simulink model "PassengerVehicle"  (R2018b)
settings: configuration reference "Physics" (kept outside this file)
model workspace (MAT data in the model file):
  m = 1000
undefined symbols (not defined in the file): activate_Banking, activate_TrackProfile, P_BrakeGain, P_PassengerVehicleSimModel, P_SimFailureRearAxleGripStepEndTime_s, P_SimFailureRearAxleGripStepTime_s, POWTR__MODE__activate_ThrottleInterface, psi_rad, tireFR__MFSIMPLE__r_tire_m, tireRL__MFSIMPLE__r_tire_m, tSPhysics, VEH__ActuatorLimitation__deltaSteering_max_rad, VEH__ActuatorLimitation__deltaSteering_min_rad, VEH__ActuatorLimitation__Fx_Brake_max_N, VEH__ActuatorLimitation__Fx_Throttle_max_N, VEH__Brakes__BrakeBias_Front, VEH__Brakes__d_BrakeActuatorBoreFrRe_m__1, VEH__Brakes__d_BrakeActuatorBoreFrRe_m__2, VEH__Brakes__mue_BrakePadsFrRe_kinetic__1, VEH__Brakes__mue_BrakePadsFrRe_kinetic__2, VEH__Brakes__n_BrakePadsNumberFrRe__1, VEH__Brakes__n_BrakePadsNumberFrRe__2, VEH__Brakes__r_BrakePadsMeanLeverFrRe_m__1, VEH__Brakes__r_BrakePadsMeanLeverFrRe_m__2, VEH__Steering__T_Steering_s, VEH__VehicleData__l_WheelbaseF_m, VEH__VehicleData__l_WheelbaseTotal_m, VEH__VehicleData__w_TrackF_m, VEH__VehicleData__w_TrackR_m, x_m, y_m
libraries: general_sensor_lib x27, simulink x12
settings Model: DataDictionary=PassengerVehicle.sldd  PauseTimes=9.280  Creator=wischnewski  LastModifiedBy=ga25xiw

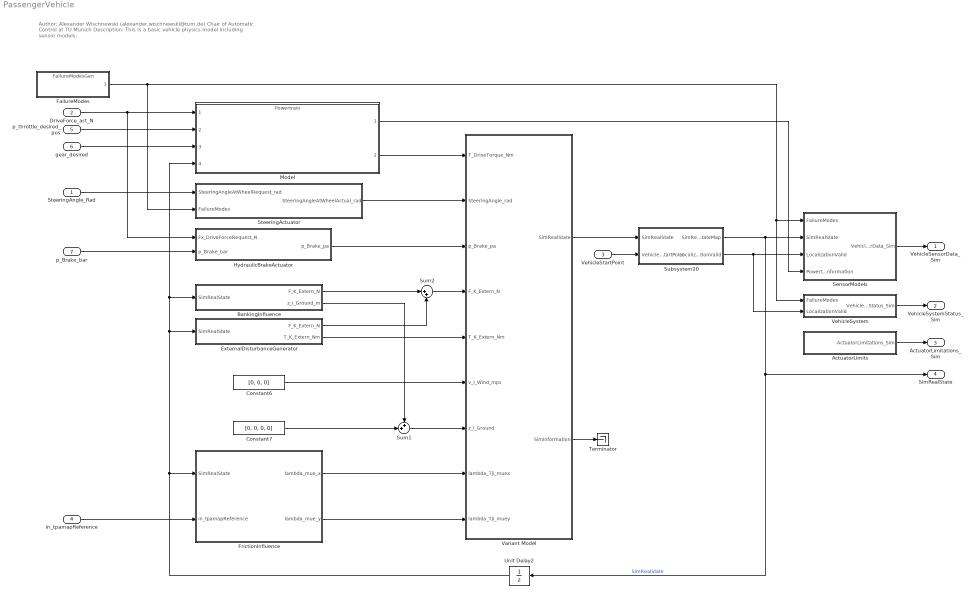
== system PassengerVehicle ==
  note: Author: Alexander Wischnewski (alexander.wischnewski@tum.de)
      | Chair of Automatic Control at TU Munich
      |
      | Description: This is a basic vehicle physics model including sensor models.
  SteeringAngle_Rad : Inport
  DriveForce_act_N : Inport  Port=2
  VehicleStartPoint : Inport  Port=3
  in_tpamapReference : Inport  Port=4  OutDataTypeStr=Bus: tpamapReference
  p_throttle_desired_pos : Inport  Port=5
  gear_desired : Inport  Port=6
  p_Brake_bar : Inport  Port=7
  ActuatorLimits : Subsystem
  BankingInfluence : Subsystem
  Constant6 : Constant  Value=[0, 0, 0]
  Constant7 : Constant  Value=[0, 0, 0, 0]
  ExternalDisturbanceGenerator : Subsystem
  FailureModes : ModelReference  ModelNameDialog=FailureModesGen  SimulationMode=Normal  ModelReferenceVersion=1.712
  FrictionInfluence : Subsystem
  HydraulicBrakeActuator : Subsystem
  Model : ModelReference  ModelNameDialog=Powertrain.slx  SimulationMode=Normal  ModelReferenceVersion=1.922
  SensorModels : Subsystem
  SteeringActuator : Subsystem
  Subsystem20 : Subsystem
  Sum1 : Sum  Inputs=++|
  Sum2 : Sum  Inputs=|++
  Terminator : Terminator
  Unit Delay2 : UnitDelay  SampleTime=-1
  Variant Model : Subsystem  Variant=on
  VehicleSystem : Subsystem
  VehicleSensorData_Sim : Outport  OutDataTypeStr=Bus: VehicleSensorData_Sim
  VehicleSystemStatus_Sim : Outport  Port=2  OutDataTypeStr=Bus: VehicleSystemStatus_Sim
  ActuatorLimitations_Sim : Outport  Port=3  OutDataTypeStr=Bus: ActuatorLimitations_Sim
  SimRealState : Outport  Port=4  OutDataTypeStr=Bus: SimRealState
  wires:
  FailureModes/1 -> SteeringActuator/2(FailureModes), VehicleSystem/1(FailureModes), SensorModels/1(FailureModes)
  SteeringActuator/1(SteeringAngleAtWheelActual_rad) -> Variant Model/2(SteeringAngle_rad)
  SensorModels/1(VehicleSensorData_Sim) -> VehicleSensorData_Sim/1
  Constant6/1 -> Variant Model/6(v_I_Wind_mps)
  VehicleSystem/1(VehicleSystemStatus_Sim) -> VehicleSystemStatus_Sim/1
  ActuatorLimits/1(ActuatorLimitations_Sim) -> ActuatorLimitations_Sim/1
  SteeringAngle_Rad/1 -> SteeringActuator/1(SteeringAngleAtWheelRequest_rad)
  HydraulicBrakeActuator/1(p_Brake_pa) -> Variant Model/3(p_Brake_pa)
  DriveForce_act_N/1 -> HydraulicBrakeActuator/1(Fx_DriveForceRequest_N), Model/1
  Model/2 -> Variant Model/1(T_DriveTorque_Nm)
  Subsystem20/1(SimRealStateMap) -> SensorModels/2(SimRealState), SimRealState/1, Unit Delay2/1  "SimRealState"
  VehicleStartPoint/1 -> Subsystem20/2(VehicleStartPoint)
  Subsystem20/2(LocalizationValid) -> VehicleSystem/2(LocalizationValid), SensorModels/3(LocalizationValid)
  Variant Model/1(SimRealState) -> Subsystem20/1(SimRealState)
  Variant Model/2(SimInformation) -> Terminator/1
  ExternalDisturbanceGenerator/2(T_K_Extern_Nm) -> Variant Model/5(T_K_Extern_Nm)
  ExternalDisturbanceGenerator/1(F_K_Extern_N) -> Sum2/2
  BankingInfluence/1(F_K_Extern_N) -> Sum2/1
  Sum2/1 -> Variant Model/4(F_K_Extern_N)
  Sum1/1 -> Variant Model/7(z_I_Ground)
  BankingInfluence/2(z_I_Ground_m) -> Sum1/1
  Constant7/1 -> Sum1/2
  FrictionInfluence/2(lambda_mue_y) -> Variant Model/9(lambda_Tji_muey)
  FrictionInfluence/1(lambda_mue_x) -> Variant Model/8(lambda_Tji_muex)
  in_tpamapReference/1 -> FrictionInfluence/2(in_tpamapReference)
  p_throttle_desired_pos/1 -> Model/2
  gear_desired/1 -> Model/3
  Model/1 -> SensorModels/4(PowertrainInformation)
  Unit Delay2/1 -> ExternalDisturbanceGenerator/1(SimRealState), Model/4, BankingInfluence/1(SimRealState), FrictionInfluence/1(SimRealState)
  p_Brake_bar/1 -> HydraulicBrakeActuator/2(p_Brake_bar)

== system PassengerVehicle/ActuatorLimits ==
  Bus Creator : BusCreator  Inputs=4  OutDataTypeStr=Bus: ActuatorLimitations_Sim
  Constant : Constant  Value=VEH__ActuatorLimitation__deltaSteering_max_rad
  Constant1 : Constant  Value=VEH__ActuatorLimitation__deltaSteering_min_rad
  Constant2 : Constant  Value=VEH__ActuatorLimitation__Fx_Throttle_max_N
  Constant3 : Constant  Value=VEH__ActuatorLimitation__Fx_Brake_max_N
  ActuatorLimitations_Sim : Outport
  wires:
  Bus Creator/1 -> ActuatorLimitations_Sim/1
  Constant/1 -> Bus Creator/1  "SteeringAngleMax_rad"
  Constant1/1 -> Bus Creator/2  "SteeringAngleMin_rad"
  Constant2/1 -> Bus Creator/3  "DriveForceMax_N"
  Constant3/1 -> Bus Creator/4  "DriveForceMin_N"

== system PassengerVehicle/BankingInfluence ==
  SimRealState : Inport  OutDataTypeStr=Bus: SimRealState
  Banking disabled : Subsystem  TreatAsAtomicUnit=on
  Banking enabled : Subsystem  TreatAsAtomicUnit=on
  Compare To Zero : simulink/Logic and Bit Operations/Compare To Zero  relop===  OutDataTypeStr=boolean
  Constant : Constant  Value=activate_Banking
  Merge : Subsystem
  F_K_Extern_N : Outport
  z_I_Ground_m : Outport  Port=2
  wires:
  SimRealState/1 -> Banking enabled/1(SimRealState), Banking disabled/1(SimRealState)
  Constant/1 -> Merge/3(In3), Compare To Zero/1, Banking enabled/Enable
  Compare To Zero/1 -> Banking disabled/Enable
  Banking enabled/1(F_K_Extern_N) -> Merge/1(In1)
  Banking enabled/2(z_I_Ground_m) -> Merge/2(In2)
  Banking disabled/1(F_K_Extern_N) -> Merge/4(In4)
  Banking disabled/2(z_I_Ground_m) -> Merge/5(In5)
  Merge/1(Out1) -> F_K_Extern_N/1
  Merge/2(Out2) -> z_I_Ground_m/1

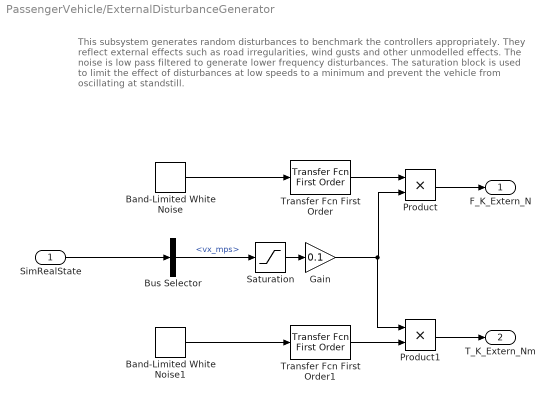
== system PassengerVehicle/ExternalDisturbanceGenerator ==
  note: This subsystem generates random disturbances to
      | benchmark the controllers appropriately. They reflect external effects
      | such as road irregularities, wind gusts and other unmodelled effects.
      |
      | The noise is low pass filtered to generate lower frequency disturbances.
      |
      | The saturation block is used to limit the effect of disturbances at low speeds to a minimum
      | and prevent the vehicle from oscillating at standstill.
  SimRealState : Inport
  Band-Limited White Noise : simulink/Sources/Band-Limited White Noise  Cov=[100^2 100^2 100^2]  Ts=tSPhysics  seed=[23341 325 10250]
  Band-Limited White Noise1 : simulink/Sources/Band-Limited White Noise  Cov=[25^2 25^2 25^2]  Ts=tSPhysics  seed=[456 7599 12475]
  Bus Selector : BusSelector  OutputSignals=vx_mps
  Gain : Gain  Gain=0.1
  Product : Product
  Product1 : Product
  Saturation : Saturate  UpperLimit=10  LowerLimit=0
  Transfer Fcn First Order : simulink/Discrete/Transfer Fcn First Order  PoleZ=0.99  ICPrevOutput=0.0  DoSatur=off
      settings: SourceProductName=Simulink
  Transfer Fcn First Order1 : simulink/Discrete/Transfer Fcn First Order  PoleZ=0.99  ICPrevOutput=0.0  DoSatur=off
      settings: SourceProductName=Simulink
  F_K_Extern_N : Outport
  T_K_Extern_Nm : Outport  Port=2
  wires:
  Band-Limited White Noise/1 -> Transfer Fcn First Order/1
  Band-Limited White Noise1/1 -> Transfer Fcn First Order1/1
  Transfer Fcn First Order/1 -> Product/1
  Product/1 -> F_K_Extern_N/1
  Transfer Fcn First Order1/1 -> Product1/2
  Product1/1 -> T_K_Extern_Nm/1
  Bus Selector/1 -> Saturation/1  "<vx_mps>"
  Saturation/1 -> Gain/1
  Gain/1 -> Product1/1, Product/2
  SimRealState/1 -> Bus Selector/1

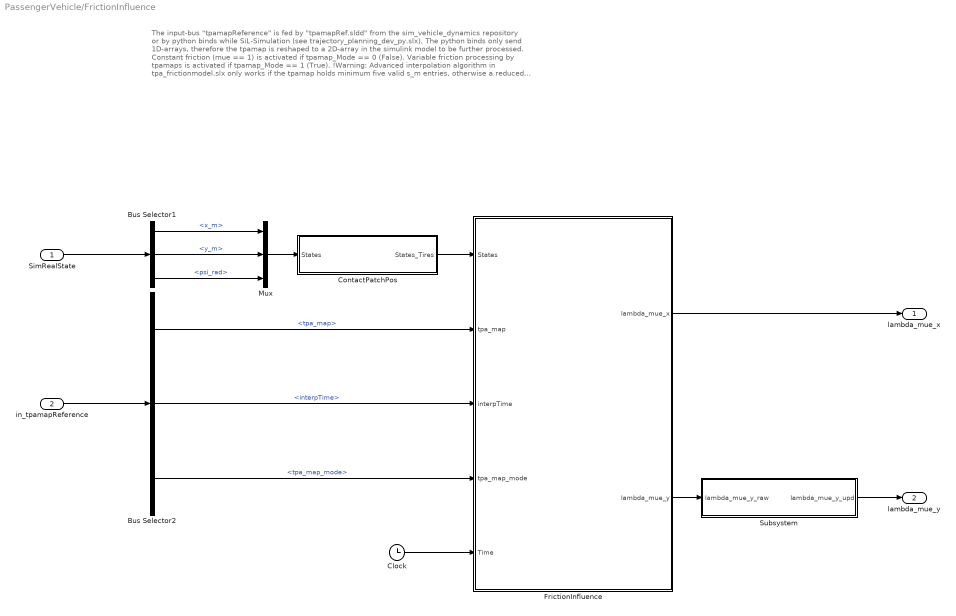
== system PassengerVehicle/FrictionInfluence ==
  note: The input-bus "tpamapReference" is fed by "tpamapRef.sldd" from the sim_vehicle_dynamics repository
      | or by python binds while SiL-Simulation (see trajectory_planning_dev_py.slx). The python binds only send
      | 1D-arrays, therefore the tpamap is reshaped to a 2D-array in the simulink model to be further processed.
      |
      | Constant friction (mue == 1) is activated if tpamap_Mode == 0 (False).
      | Variable friction processing by tpamaps is activated if tpamap_Mode == 1 (True).
      |
      | !Warning: Advanced interpolation algorithm in tpa_frictionmodel.slx only works if the tpamap holds minimum five valid s_m entries,
      |                 otherwise a reduced algorithm takes over, which assigns the local scaling factor of the nearest s_m entry to the lambda_mues
      |
      | Author: Dominik Stärk (dominik.staerk@tum.de)
  SimRealState : Inport
  in_tpamapReference : Inport  Port=2
  Bus Selector1 : BusSelector  OutputSignals=x_m,y_m,psi_rad
  Bus Selector2 : BusSelector  OutputSignals=tpa_map,interpTime,tpa_map_mode
  Clock : Clock
  ContactPatchPos : MATLAB Function  TreatAsAtomicUnit=on
  FrictionInfluence : MATLAB Function  TreatAsAtomicUnit=on
  Mux : Mux  Inputs=3
  Subsystem : Subsystem
  lambda_mue_x : Outport
  lambda_mue_y : Outport  Port=2
  wires:
  Bus Selector1/1 -> Mux/1  "<x_m>"
  Bus Selector1/2 -> Mux/2  "<y_m>"
  in_tpamapReference/1 -> Bus Selector2/1
  SimRealState/1 -> Bus Selector1/1
  Clock/1 -> FrictionInfluence/5(Time)
  Mux/1 -> ContactPatchPos/1(States)
  Bus Selector2/1 -> FrictionInfluence/2(tpa_map)  "<tpa_map>"
  Bus Selector2/2 -> FrictionInfluence/3(interpTime)  "<interpTime>"
  Bus Selector2/3 -> FrictionInfluence/4(tpa_map_mode)  "<tpa_map_mode>"
  FrictionInfluence/1(lambda_mue_x) -> lambda_mue_x/1
  Bus Selector1/3 -> Mux/3  "<psi_rad>"
  ContactPatchPos/1(States_Tires) -> FrictionInfluence/1(States)
  FrictionInfluence/2(lambda_mue_y) -> Subsystem/1(lambda_mue_y_raw)
  Subsystem/1(lambda_mue_y_upd) -> lambda_mue_y/1

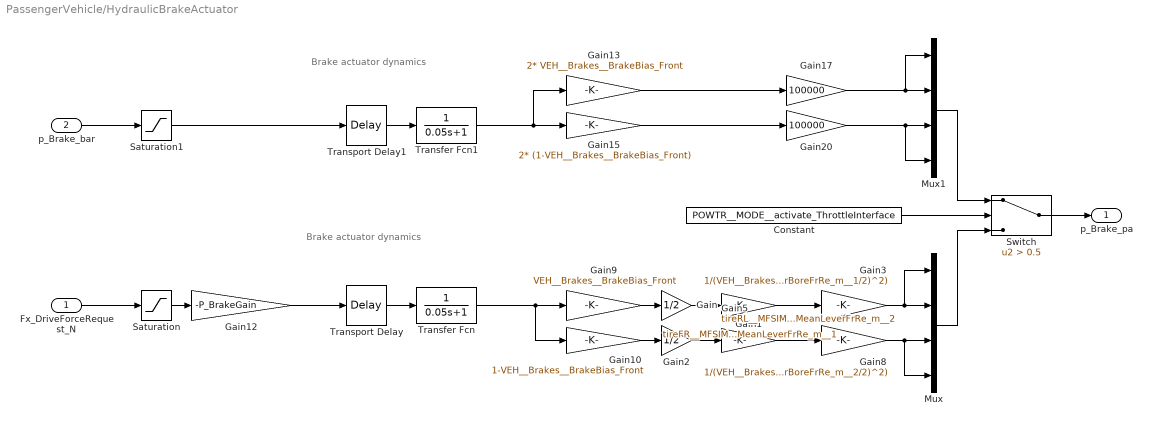
== system PassengerVehicle/HydraulicBrakeActuator ==
  note: Brake actuator dynamics
  note: Brake actuator dynamics
  Fx_DriveForceRequest_N : Inport
  p_Brake_bar : Inport  Port=2
  Constant : Constant  Value=POWTR__MODE__activate_ThrottleInterface
  Gain : Gain  Gain=1/2
  Gain1 : Gain  Gain=tireFR__MFSIMPLE__r_tire_m / VEH__Brakes__r_BrakePadsMeanLeverFrRe_m__1
  Gain10 : Gain  Gain=1-VEH__Brakes__BrakeBias_Front
  Gain12 : Gain  Gain=-P_BrakeGain
  Gain13 : Gain  Gain=2* VEH__Brakes__BrakeBias_Front
  Gain15 : Gain  Gain=2* (1-VEH__Brakes__BrakeBias_Front)
  Gain17 : Gain  Gain=100000
  Gain2 : Gain  Gain=1/2
  Gain20 : Gain  Gain=100000
  Gain3 : Gain  Gain=1/(VEH__Brakes__n_BrakePadsNumberFrRe__1*VEH__Brakes__mue_BrakePadsFrRe_kinetic__1*pi*(VEH__Brakes__d_BrakeActuatorBoreFrRe_m__1/2)^2)
  Gain5 : Gain  Gain=tireRL__MFSIMPLE__r_tire_m / VEH__Brakes__r_BrakePadsMeanLeverFrRe_m__2
  Gain8 : Gain  Gain=1/(VEH__Brakes__n_BrakePadsNumberFrRe__2*VEH__Brakes__mue_BrakePadsFrRe_kinetic__2*pi*(VEH__Brakes__d_BrakeActuatorBoreFrRe_m__2/2)^2)
  Gain9 : Gain  Gain=VEH__Brakes__BrakeBias_Front
  Mux : Mux
  Mux1 : Mux
  Saturation : Saturate  UpperLimit=0  LowerLimit=-inf
  Saturation1 : Saturate  UpperLimit=inf  LowerLimit=0
  Switch : Switch  Criteria=u2 > Threshold  Threshold=0.5
  Transfer Fcn : TransferFcn  Denominator=[0.05 1]
  Transfer Fcn1 : TransferFcn  Denominator=[0.05 1]
  Transport Delay : TransportDelay  DelayTime=0.02
  Transport Delay1 : TransportDelay  DelayTime=0.02
  p_Brake_pa : Outport
  wires:
  Gain8/1 -> Mux/3, Mux/4
  Gain3/1 -> Mux/1, Mux/2
  Fx_DriveForceRequest_N/1 -> Saturation/1
  Transfer Fcn/1 -> Gain10/1, Gain9/1
  Gain5/1 -> Gain8/1
  Gain1/1 -> Gain3/1
  Saturation/1 -> Gain12/1
  Transport Delay/1 -> Transfer Fcn/1
  Gain12/1 -> Transport Delay/1
  Constant/1 -> Switch/2
  p_Brake_bar/1 -> Saturation1/1
  Transport Delay1/1 -> Transfer Fcn1/1
  Saturation1/1 -> Transport Delay1/1
  Transfer Fcn1/1 -> Gain13/1, Gain15/1
  Gain13/1 -> Gain17/1
  Gain15/1 -> Gain20/1
  Mux1/1 -> Switch/1
  Mux/1 -> Switch/3
  Switch/1 -> p_Brake_pa/1
  Gain17/1 -> Mux1/1, Mux1/2
  Gain20/1 -> Mux1/4, Mux1/3
  Gain9/1 -> Gain/1
  Gain/1 -> Gain1/1
  Gain10/1 -> Gain2/1
  Gain2/1 -> Gain5/1

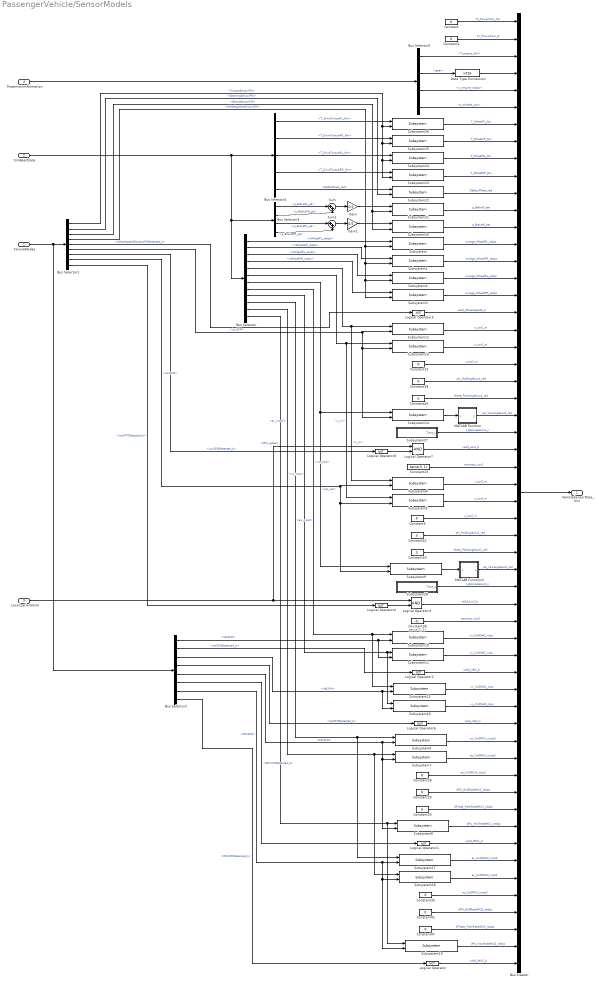
== system PassengerVehicle/SensorModels ==
  FailureModes : Inport
  SimRealState : Inport  Port=2
  LocalizationValid : Inport  Port=3
  PowertrainInformation : Inport  Port=4
  Bus Creator : BusCreator  Inputs=56  OutDataTypeStr=Bus: VehicleSensorData_Sim
  Bus Selector : BusSelector  OutputSignals=nWheelFL_radps,nWheelFR_radps,nWheelRL_radps,nWheelRR_radps,x_m,y_m,psi_rad,vx_mps,vy_mps,ax_mps2,ay_mps2,dPsi_radps
  Bus Selector1 : BusSelector  OutputSignals=TorqueSensorFM,SteeringSensorFM,BrakeSensorFM,WheelspeedSensorsFM,WheelspeedSensorsFMDetected_b,Loc1FM,Loc1FMDetected_b,Loc2FM,Loc2FMDetected_b
  Bus Selector2 : BusSelector  OutputSignals=Vel1FM,Vel1FMDetected_b,Vel2FM,Vel2FMDetected_b,IMU1FM,IMU1FMDetected_b,IMU2FM,IMU2FMDetected_b
  Bus Selector3 : BusSelector  OutputSignals=p_BrakeFL_pa,p_BrakeFR_pa,p_BrakeRL_pa,p_BrakeRR_pa
  Bus Selector4 : BusSelector  OutputSignals=T_DriveTorqueFL_Nm,T_DriveTorqueFR_Nm,T_DriveTorqueRL_Nm,T_DriveTorqueRR_Nm,DeltaWheel_rad
  Bus Selector5 : BusSelector  OutputSignals=T_engine_Nm,gear,w_engine_radps,p_throttle_pos
  Constant{,1,6,15,28..30,35,39..43,47} (14 alike) : Constant  Value=0
  Constant23 : Constant  Value=zeros(3, 1)
  Constant38 : Constant  Value=zeros(3, 1)
  Data Type Conversion : DataTypeConversion  OutDataTypeStr=int16
  Gain : Gain  Gain=0.5
  Gain1 : Gain  Gain=0.5
  Logical Operator{,1..2,4..6,8} (7 alike) : Logic  Operator=NOT  Inputs=1  AllPortsSameDT=off  OutDataTypeStr=boolean
  Logical Operator3 : Logic  AllPortsSameDT=off  OutDataTypeStr=boolean
  Logical Operator7 : Logic  AllPortsSameDT=off  OutDataTypeStr=boolean
  MATLAB Function : MATLAB Function  TreatAsAtomicUnit=on
  MATLAB Function2 : MATLAB Function  TreatAsAtomicUnit=on
  Subsystem : general_sensor_lib/Subsystem  Noise=0.1  Delay=0  SampleRate=tSPhysics  seed=436
  Subsystem1 : general_sensor_lib/Subsystem  Noise=0.1  Delay=0  SampleRate=tSPhysics  seed=438
  Subsystem10 : general_sensor_lib/Subsystem  Noise=0.01  Delay=0  SampleRate=tSPhysics  seed=4577
  Subsystem11 : general_sensor_lib/Subsystem  Noise=0.01  Delay=0  SampleRate=tSPhysics  seed=127
  Subsystem12 : general_sensor_lib/Subsystem  Noise=0.001  Delay=0  SampleRate=tSPhysics  seed=596
  Subsystem13 : general_sensor_lib/Subsystem  Noise=0.001  Delay=0  SampleRate=tSPhysics  seed=973
  Subsystem14 : general_sensor_lib/Subsystem  Noise=0.001  Delay=0  SampleRate=tSPhysics  seed=578
  Subsystem15 : general_sensor_lib/Subsystem  Noise=0.01  Delay=0  SampleRate=tSPhysics  seed=459
  Subsystem16 : general_sensor_lib/Subsystem  Noise=0.01  Delay=0  SampleRate=tSPhysics  seed=467
  Subsystem17 : general_sensor_lib/Subsystem  Noise=0.05  Delay=0  SampleRate=tSPhysics  seed=37
  Subsystem18 : general_sensor_lib/Subsystem  Noise=0.05  Delay=0  SampleRate=tSPhysics  seed=0
  Subsystem19 : general_sensor_lib/Subsystem  Noise=0.0002  Delay=0  SampleRate=tSPhysics  seed=0
  Subsystem2 : general_sensor_lib/Subsystem  Noise=0.1  Delay=0  SampleRate=tSPhysics  seed=137
  Subsystem20 : general_sensor_lib/Subsystem  Noise=1000000000  Delay=0  SampleRate=tSPhysics  seed=235
  Subsystem21 : general_sensor_lib/Subsystem  Noise=1000000000  Delay=0  SampleRate=tSPhysics  seed=798
  Subsystem22 : general_sensor_lib/Subsystem  Noise=1e-7  Delay=0  SampleRate=tSPhysics  seed=1234
  Subsystem23 : general_sensor_lib/Subsystem  Noise=100  Delay=0  SampleRate=tSPhysics  seed=438
  Subsystem24 : general_sensor_lib/Subsystem  Noise=100  Delay=0  SampleRate=tSPhysics  seed=368
  Subsystem25 : general_sensor_lib/Subsystem  Noise=100  Delay=0  SampleRate=tSPhysics  seed=978
  Subsystem26 : general_sensor_lib/Subsystem  Noise=100  Delay=0  SampleRate=tSPhysics  seed=138
  Subsystem27 : Subsystem
  Subsystem28 : Subsystem
  Subsystem3 : general_sensor_lib/Subsystem  Noise=0.1  Delay=0  SampleRate=tSPhysics  seed=345
  Subsystem4 : general_sensor_lib/Subsystem  Noise=0.001  Delay=0  SampleRate=tSPhysics  seed=596
  Subsystem5 : general_sensor_lib/Subsystem  Noise=0.001  Delay=0  SampleRate=tSPhysics  seed=973
  Subsystem6 : general_sensor_lib/Subsystem  Noise=0.05  Delay=0  SampleRate=tSPhysics  seed=456
  Subsystem7 : general_sensor_lib/Subsystem  Noise=0.05  Delay=0  SampleRate=tSPhysics  seed=78
  Subsystem8 : general_sensor_lib/Subsystem  Noise=0.0002  Delay=0  SampleRate=tSPhysics  seed=43
  Subsystem9 : general_sensor_lib/Subsystem  Noise=0.001  Delay=0  SampleRate=tSPhysics  seed=578
  Sum : Sum  Inputs=|++
  Sum1 : Sum  Inputs=|++
  VehicleSensorData_Sim : Outport
  wires:
  Bus Creator/1 -> VehicleSensorData_Sim/1
  Constant/1 -> Bus Creator/1  "Tz_Powertrain_Nm"
  Constant1/1 -> Bus Creator/2  "Fx_Powertrain_N"
  SimRealState/1 -> Bus Selector/1, Bus Selector3/1, Bus Selector4/1
  Bus Selector/1 -> Subsystem/1  "<nWheelFL_radps>"
  Bus Selector/2 -> Subsystem1/1  "<nWheelFR_radps>"
  Bus Selector/3 -> Subsystem2/1  "<nWheelRL_radps>"
  Bus Selector/4 -> Subsystem3/1  "<nWheelRR_radps>"
  Bus Selector/5 -> Subsystem4/1, Subsystem12/1  "<x_m>"
  Bus Selector/6 -> Subsystem5/1, Subsystem13/1  "<y_m>"
  Bus Selector/10 -> Subsystem17/1, Subsystem6/1  "<ax_mps2>"
  Bus Selector/11 -> Subsystem7/1, Subsystem18/1  "<ay_mps2>"
  Bus Selector/12 -> Subsystem19/1, Subsystem8/1  "<dPsi_radps>"
  Bus Selector/8 -> Subsystem15/1, Subsystem10/1  "<vx_mps>"
  Bus Selector/9 -> Subsystem16/1, Subsystem11/1  "<vy_mps>"
  Bus Selector/7 -> Subsystem9/1, Subsystem14/1  "<psi_rad>"
  FailureModes/1 -> Bus Selector1/1, Bus Selector2/1
  Bus Selector1/4 -> Subsystem/2, Subsystem1/2, Subsystem2/2, Subsystem3/2  "<WheelspeedSensorsFM>"
  Bus Selector1/5 -> Logical Operator5/1  "<WheelspeedSensorsFMDetected_b>"
  Bus Selector2/1 -> Subsystem11/2, Subsystem10/2  "<Vel1FM>"
  Bus Selector2/2 -> Logical Operator2/1  "<Vel1FMDetected_b>"
  Bus Selector2/5 -> Subsystem8/2, Subsystem7/2, Subsystem6/2  "<IMU1FM>"
  Bus Selector2/6 -> Logical Operator1/1  "<IMU1FMDetected_b>"
  Subsystem9/1 -> MATLAB Function2/1(u)
  Bus Selector2/3 -> Subsystem16/2, Subsystem15/2  "<Vel2FM>"
  Bus Selector2/4 -> Logical Operator6/1  "<Vel2FMDetected_b>"
  Bus Selector2/7 -> Subsystem19/2, Subsystem18/2, Subsystem17/2  "<IMU2FM>"
  Bus Selector2/8 -> Logical Operator/1  "<IMU2FMDetected_b>"
  Subsystem14/1 -> MATLAB Function/1(u)
  Logical Operator4/1 -> Logical Operator3/2
  Bus Selector1/9 -> Logical Operator4/1  "<Loc2FMDetected_b>"
  LocalizationValid/1 -> Logical Operator7/1, Logical Operator3/1
  Bus Selector1/8 -> Subsystem9/2, Subsystem5/2, Subsystem4/2  "<Loc2FM>"
  Bus Selector1/6 -> Subsystem14/2, Subsystem13/2, Subsystem12/2  "<Loc1FM>"
  Logical Operator8/1 -> Logical Operator7/2
  Bus Selector1/7 -> Logical Operator8/1  "<Loc1FMDetected_b>"
  Sum/1 -> Gain/1
  Sum1/1 -> Gain1/1
  Gain1/1 -> Subsystem20/1
  Gain/1 -> Subsystem21/1
  Bus Selector4/1 -> Subsystem26/1  "<T_DriveTorqueFL_Nm>"
  Bus Selector4/2 -> Subsystem25/1  "<T_DriveTorqueFR_Nm>"
  Bus Selector4/5 -> Subsystem22/1  "<DeltaWheel_rad>"
  Bus Selector3/1 -> Sum/1  "<p_BrakeFL_pa>"
  Bus Selector3/3 -> Sum1/1  "<p_BrakeRL_pa>"
  Bus Selector3/2 -> Sum/2  "<p_BrakeFR_pa>"
  Bus Selector3/4 -> Sum1/2  "<p_BrakeRR_pa>"
  Bus Selector4/4 -> Subsystem23/1  "<T_DriveTorqueRR_Nm>"
  Bus Selector4/3 -> Subsystem24/1  "<T_DriveTorqueRL_Nm>"
  Bus Selector1/3 -> Subsystem21/2, Subsystem20/2  "<BrakeSensorFM>"
  Bus Selector1/2 -> Subsystem22/2  "<SteeringSensorFM>"
  Bus Selector1/1 -> Subsystem23/2, Subsystem24/2, Subsystem25/2, Subsystem26/2  "<TorqueSensorFM>"
  PowertrainInformation/1 -> Bus Selector5/1
  Bus Selector5/1 -> Bus Creator/3  "<T_engine_Nm>"
  Bus Selector5/2 -> Data Type Conversion/1  "<gear>"
  Bus Selector5/3 -> Bus Creator/5  "<w_engine_radps>"
  Bus Selector5/4 -> Bus Creator/6  "<p_throttle_pos>"
  Subsystem26/1 -> Bus Creator/7  "T_WheelFL_Nm"
  Subsystem25/1 -> Bus Creator/8  "T_WheelFR_Nm"
  Subsystem24/1 -> Bus Creator/9  "T_WheelRL_Nm"
  Subsystem23/1 -> Bus Creator/10  "T_WheelRR_Nm"
  Subsystem22/1 -> Bus Creator/11  "Delta_Wheel_rad"
  Subsystem20/1 -> Bus Creator/13  "p_BrakeR_bar"
  Subsystem21/1 -> Bus Creator/12  "p_BrakeF_bar"
  Subsystem/1 -> Bus Creator/14  "omega_WheelFL_radps"
  Subsystem1/1 -> Bus Creator/15  "omega_WheelFR_radps"
  Subsystem2/1 -> Bus Creator/16  "omega_WheelRL_radps"
  Subsystem3/1 -> Bus Creator/17  "omega_WheelRR_radps"
  Logical Operator5/1 -> Bus Creator/18  "valid_Wheelspeeds_b"
  Subsystem12/1 -> Bus Creator/19  "x_Loc1_m"
  Subsystem13/1 -> Bus Creator/20  "y_Loc1_m"
  Constant15/1 -> Bus Creator/21  "z_Loc1_m"
  Constant39/1 -> Bus Creator/22  "phi_RollAngleLoc1_rad"
  Constant40/1 -> Bus Creator/23  "theta_PitchAngleLoc1_rad"
  MATLAB Function/1(y) -> Bus Creator/24  "psi_YawAngleLoc1_rad"
  Subsystem27/1(Time_s) -> Bus Creator/25  "t_EstimateLoc1_s"
  Logical Operator7/1 -> Bus Creator/26  "valid_Loc1_b"
  Constant23/1 -> Bus Creator/27  "accuracy_Loc1"
  Constant6/1 -> Bus Creator/30  "z_Loc2_m"
  Constant42/1 -> Bus Creator/31  "phi_RollAngleLoc2_rad"
  Constant43/1 -> Bus Creator/32  "theta_PitchAngleLoc2_rad"
  Subsystem5/1 -> Bus Creator/29  "y_Loc2_m"
  Subsystem4/1 -> Bus Creator/28  "x_Loc2_m"
  MATLAB Function2/1(y) -> Bus Creator/33  "psi_YawAngleLoc2_rad"
  Subsystem28/1(Time_s) -> Bus Creator/34  "t_EstimateLoc2_s"
  Logical Operator3/1 -> Bus Creator/35  "valid_Loc2_b"
  Constant38/1 -> Bus Creator/36  "accuracy_Loc2"
  Subsystem10/1 -> Bus Creator/37  "vx_CoGVel1_mps"
  Subsystem11/1 -> Bus Creator/38  "vy_CoGVel1_mps"
  Logical Operator2/1 -> Bus Creator/39  "valid_Vel1_b"
  Subsystem15/1 -> Bus Creator/40  "vx_CoGVel2_mps"
  Subsystem16/1 -> Bus Creator/41  "vy_CoGVel2_mps"
  Logical Operator6/1 -> Bus Creator/42  "valid_Vel2_b"
  Subsystem6/1 -> Bus Creator/43  "ax_CoGIMU1_mps2"
  Subsystem7/1 -> Bus Creator/44  "ay_CoGIMU1_mps2"
  Constant28/1 -> Bus Creator/45  "az_CoGIMU1_mps2"
  Constant29/1 -> Bus Creator/46  "dPhi_RollRateIMU1_radps"
  Constant30/1 -> Bus Creator/47  "dTheta_PitchRateIMU1_radps"
  Subsystem8/1 -> Bus Creator/48  "dPsi_YawRateIMU1_radps"
  Logical Operator1/1 -> Bus Creator/49  "valid_IMU1_b"
  Subsystem17/1 -> Bus Creator/50  "ax_CoGIMU2_mps2"
  Subsystem18/1 -> Bus Creator/51  "ay_CoGIMU2_mps2"
  Constant35/1 -> Bus Creator/52  "az_CoGIMU2_mps2"
  Constant41/1 -> Bus Creator/53  "dPhi_RollRateIMU2_radps"
  Constant47/1 -> Bus Creator/54  "dTheta_PitchRateIMU2_radps"
  Subsystem19/1 -> Bus Creator/55  "dPsi_YawRateIMU2_radps"
  Logical Operator/1 -> Bus Creator/56  "valid_IMU2_b"
  Data Type Conversion/1 -> Bus Creator/4

== system PassengerVehicle/SteeringActuator ==
  SteeringAngleAtWheelRequest_rad : Inport
  FailureModes : Inport  Port=2
  Bus Selector : BusSelector  OutputSignals=SteeringActuatorFM
  Switch : Switch  Criteria=u2 > Threshold
  Transfer Fcn : TransferFcn  Denominator=[VEH__Steering__T_Steering_s 1]
  Unit Delay : UnitDelay  SampleTime=-1
  SteeringAngleAtWheelActual_rad : Outport
  wires:
  Unit Delay/1 -> Switch/1
  Switch/1 -> Transfer Fcn/1, Unit Delay/1
  SteeringAngleAtWheelRequest_rad/1 -> Switch/3
  FailureModes/1 -> Bus Selector/1
  Bus Selector/1 -> Switch/2  "<SteeringActuatorFM>"
  Transfer Fcn/1 -> SteeringAngleAtWheelActual_rad/1

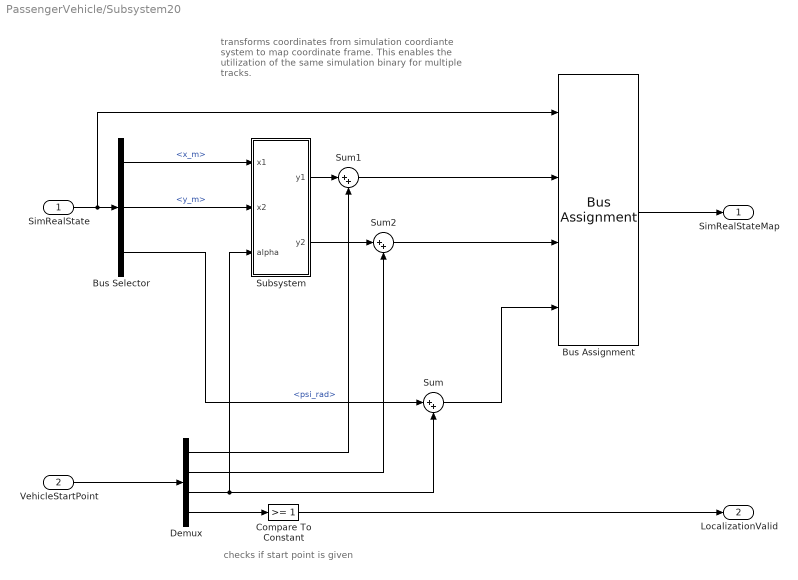
== system PassengerVehicle/Subsystem20 ==
  note: transforms coordinates from simulation
      | coordiante system to map coordinate frame.
      | This enables the utilization of the same simulation
      | binary for multiple tracks.
  note: checks if start point is given
  SimRealState : Inport
  VehicleStartPoint : Inport  Port=2
  Bus Assignment : BusAssignment  AssignedSignals=x_m,y_m,psi_rad
  Bus Selector : BusSelector  OutputSignals=x_m,y_m,psi_rad
  Compare To Constant : simulink/Logic and Bit Operations/Compare To Constant  relop=>=  const=1  OutDataTypeStr=boolean
  Demux : Demux
  Subsystem : Subsystem
  Sum : Sum  Inputs=|++
  Sum1 : Sum  Inputs=|++
  Sum2 : Sum  Inputs=|++
  SimRealStateMap : Outport
  LocalizationValid : Outport  Port=2
  wires:
  VehicleStartPoint/1 -> Demux/1
  Demux/4 -> Compare To Constant/1
  Bus Selector/2 -> Subsystem/2(x2)  "<y_m>"
  Bus Selector/1 -> Subsystem/1(x1)  "<x_m>"
  Demux/3 -> Sum/2, Subsystem/3(alpha)
  Bus Selector/3 -> Sum/1  "<psi_rad>"
  Demux/1 -> Sum1/2
  Subsystem/2(y2) -> Sum2/1
  Demux/2 -> Sum2/2
  SimRealState/1 -> Bus Assignment/1, Bus Selector/1
  Compare To Constant/1 -> LocalizationValid/1
  Subsystem/1(y1) -> Sum1/1
  Sum1/1 -> Bus Assignment/2
  Sum2/1 -> Bus Assignment/3
  Sum/1 -> Bus Assignment/4
  Bus Assignment/1 -> SimRealStateMap/1

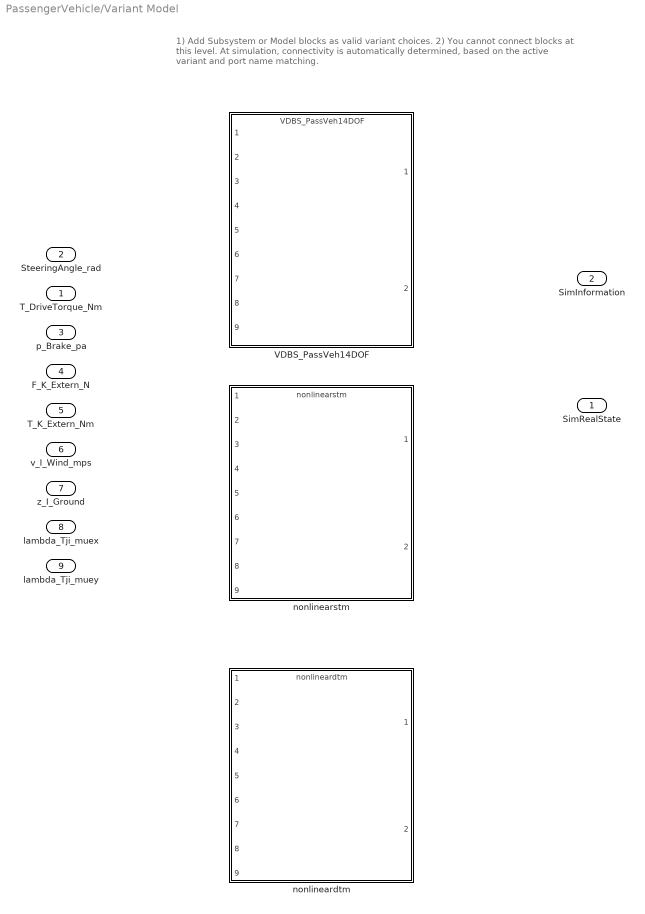
== system PassengerVehicle/Variant Model ==
  note: 1) Add Subsystem or Model blocks as valid variant choices.
      | 2) You cannot connect blocks at this level. At simulation, connectivity is automatically
      | determined, based on the active variant and port name matching.
  T_DriveTorque_Nm : Inport
  SteeringAngle_rad : Inport  Port=2
  p_Brake_pa : Inport  Port=3
  F_K_Extern_N : Inport  Port=4  PortDimensions=3
  T_K_Extern_Nm : Inport  Port=5  PortDimensions=3
  v_I_Wind_mps : Inport  Port=6  PortDimensions=3
  z_I_Ground : Inport  Port=7  PortDimensions=4
  lambda_Tji_muex : Inport  Port=8  PortDimensions=4
  lambda_Tji_muey : Inport  Port=9  PortDimensions=4
  VDBS_PassVeh14DOF : ModelReference  DisableCoverage=on  ModelNameDialog=VDBS_PassVeh14DOF.slx  SimulationMode=Normal  VariantControl=P_PassengerVehicleSimModel==3  ModelReferenceVersion=1.286
  nonlineardtm : ModelReference  ModelNameDialog=nonlineardtm.slx  ParameterArgumentNames=x0_initialstates  ParameterArgumentValues=[0 0 0 0 0 -pi/2]  UsingDefaultArgumentValue=0  SimulationMode=Normal  VariantControl=P_PassengerVehicleSimModel==2  ModelReferenceVersion=1.737
  nonlinearstm : ModelReference  ModelNameDialog=nonlinearstm  ParameterArgumentNames=x0_positionstates  ParameterArgumentValues=[0,0,0]  UsingDefaultArgumentValue=0  SimulationMode=Normal  VariantControl=P_PassengerVehicleSimModel==1  ModelReferenceVersion=1.404
  SimRealState : Outport  OutDataTypeStr=Bus: SimRealState
  SimInformation : Outport  Port=2  OutDataTypeStr=Bus: SimInformation

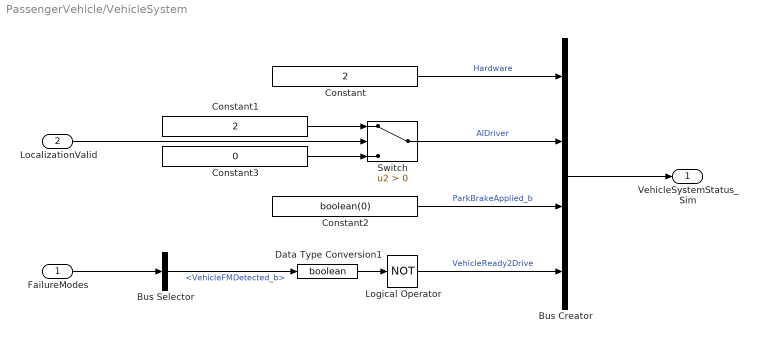
== system PassengerVehicle/VehicleSystem ==
  FailureModes : Inport
  LocalizationValid : Inport  Port=2
  Bus Creator : BusCreator  Inputs=4  OutDataTypeStr=Bus: VehicleSystemStatus_Sim
  Bus Selector : BusSelector  OutputSignals=VehicleFMDetected_b
  Constant : Constant  Value=2
  Constant1 : Constant  Value=2
  Constant2 : Constant  Value=boolean(0)
  Constant3 : Constant  Value=0
  Data Type Conversion1 : DataTypeConversion  OutDataTypeStr=boolean
  Logical Operator : Logic  Operator=NOT  Inputs=1  AllPortsSameDT=off  OutDataTypeStr=boolean
  Switch : Switch  Criteria=u2 > Threshold
  VehicleSystemStatus_Sim : Outport
  wires:
  Bus Creator/1 -> VehicleSystemStatus_Sim/1
  Constant/1 -> Bus Creator/1  "Hardware"
  Switch/1 -> Bus Creator/2  "AIDriver"
  Constant2/1 -> Bus Creator/3  "ParkBrakeApplied_b"
  Logical Operator/1 -> Bus Creator/4  "VehicleReady2Drive"
  Data Type Conversion1/1 -> Logical Operator/1
  FailureModes/1 -> Bus Selector/1
  Bus Selector/1 -> Data Type Conversion1/1  "<VehicleFMDetected_b>"
  LocalizationValid/1 -> Switch/2
  Constant1/1 -> Switch/1
  Constant3/1 -> Switch/3

== system PassengerVehicle/BankingInfluence/Banking disabled ==
  SimRealState : Inport  OutDataTypeStr=Bus: SimRealState
  Enable : EnablePort
  Constant : Constant  Value=[0 0 0]
  Constant1 : Constant  Value=[0 0 0 0]
  Terminator : Terminator
  F_K_Extern_N : Outport
  z_I_Ground_m : Outport  Port=2
  wires:
  SimRealState/1 -> Terminator/1
  Constant1/1 -> z_I_Ground_m/1
  Constant/1 -> F_K_Extern_N/1

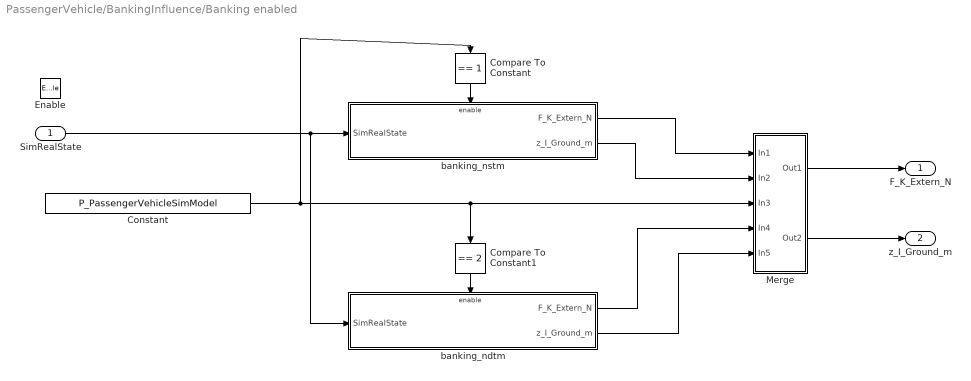
== system PassengerVehicle/BankingInfluence/Banking enabled ==
  SimRealState : Inport  OutDataTypeStr=Bus: SimRealState
  Enable : EnablePort
  Compare To Constant : simulink/Logic and Bit Operations/Compare To Constant  relop===  const=1  OutDataTypeStr=boolean
  Compare To Constant1 : simulink/Logic and Bit Operations/Compare To Constant  relop===  const=2  OutDataTypeStr=boolean
  Constant : Constant  Value=P_PassengerVehicleSimModel
  Merge : Subsystem
  banking_ndtm : Subsystem  TreatAsAtomicUnit=on
  banking_nstm : Subsystem  TreatAsAtomicUnit=on
  F_K_Extern_N : Outport
  z_I_Ground_m : Outport  Port=2
  wires:
  Compare To Constant/1 -> banking_nstm/Enable
  SimRealState/1 -> banking_ndtm/1(SimRealState), banking_nstm/1(SimRealState)
  Constant/1 -> Compare To Constant1/1, Merge/3(In3), Compare To Constant/1
  Compare To Constant1/1 -> banking_ndtm/Enable
  banking_nstm/1(F_K_Extern_N) -> Merge/1(In1)
  banking_nstm/2(z_I_Ground_m) -> Merge/2(In2)
  banking_ndtm/1(F_K_Extern_N) -> Merge/4(In4)
  banking_ndtm/2(z_I_Ground_m) -> Merge/5(In5)
  Merge/1(Out1) -> F_K_Extern_N/1
  Merge/2(Out2) -> z_I_Ground_m/1

== system PassengerVehicle/BankingInfluence/Merge ==
  In1 : Inport
  In2 : Inport  Port=2
  In3 : Inport  Port=3
  In4 : Inport  Port=4
  In5 : Inport  Port=5
  Switch : Switch  Criteria=u2 > Threshold
  Switch2 : Switch  Criteria=u2 > Threshold
  Out1 : Outport
  Out2 : Outport  Port=2
  wires:
  In2/1 -> Switch/1
  In3/1 -> Switch/2, Switch2/2
  In5/1 -> Switch/3
  Switch/1 -> Out2/1
  Switch2/1 -> Out1/1
  In4/1 -> Switch2/3
  In1/1 -> Switch2/1

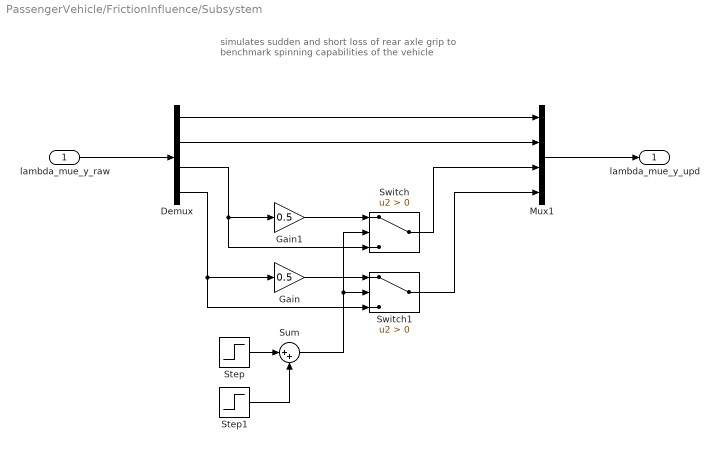
== system PassengerVehicle/FrictionInfluence/Subsystem ==
  note: simulates sudden and short loss of rear axle grip
      | to benchmark spinning capabilities of the vehicle
  lambda_mue_y_raw : Inport
  Demux : Demux
  Gain : Gain  Gain=0.5
  Gain1 : Gain  Gain=0.5
  Mux1 : Mux
  Step : Step  Time=P_SimFailureRearAxleGripStepTime_s
  Step1 : Step  Time=P_SimFailureRearAxleGripStepEndTime_s  After=-1
  Sum : Sum  Inputs=|++
  Switch : Switch  Criteria=u2 > Threshold
  Switch1 : Switch  Criteria=u2 > Threshold
  lambda_mue_y_upd : Outport
  wires:
  Sum/1 -> Switch1/2, Switch/2
  Demux/3 -> Gain1/1, Switch/3
  Step/1 -> Sum/1
  Switch/1 -> Mux1/3
  Demux/4 -> Switch1/3, Gain/1
  Step1/1 -> Sum/2
  Switch1/1 -> Mux1/4
  Gain1/1 -> Switch/1
  Gain/1 -> Switch1/1
  Demux/2 -> Mux1/2
  Demux/1 -> Mux1/1
  Mux1/1 -> lambda_mue_y_upd/1
  lambda_mue_y_raw/1 -> Demux/1

== system PassengerVehicle/SensorModels/Subsystem27 ==
  note: Own implementation necessary
      | as there are problems with codegen
      | for limited counter
  Constant2 : Constant  Value=0
  Constant3 : Constant  Value=tSPhysics
  Sum2 : Sum  Inputs=|++
  Switch : Switch  Criteria=u2 > Threshold  Threshold=0.2
  Unit Delay : UnitDelay  SampleTime=-1
  Time_s : Outport
  wires:
  Sum2/1 -> Unit Delay/1
  Unit Delay/1 -> Time_s/1, Switch/3, Switch/2
  Constant2/1 -> Switch/1
  Switch/1 -> Sum2/2
  Constant3/1 -> Sum2/1

== system PassengerVehicle/SensorModels/Subsystem28 ==
  note: Own implementation necessary
      | as there are problems with codegen
      | for limited counter
  Constant2 : Constant  Value=0
  Constant3 : Constant  Value=tSPhysics
  Sum2 : Sum  Inputs=|++
  Switch : Switch  Criteria=u2 > Threshold  Threshold=0.2
  Unit Delay : UnitDelay  SampleTime=-1
  Time_s : Outport
  wires:
  Sum2/1 -> Unit Delay/1
  Unit Delay/1 -> Time_s/1, Switch/3, Switch/2
  Constant2/1 -> Switch/1
  Switch/1 -> Sum2/2
  Constant3/1 -> Sum2/1

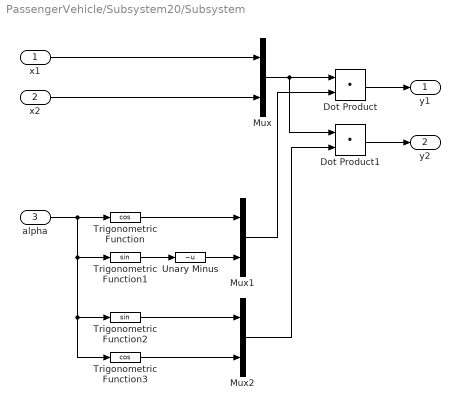
== system PassengerVehicle/Subsystem20/Subsystem ==
  x1 : Inport
  x2 : Inport  Port=2
  alpha : Inport  Port=3
  Dot Product : DotProduct  InputSameDT=on  OutDataTypeStr=Inherit: Inherit via internal rule
  Dot Product1 : DotProduct  InputSameDT=on  OutDataTypeStr=Inherit: Inherit via internal rule
  Mux : Mux  Inputs=2
  Mux1 : Mux  Inputs=2
  Mux2 : Mux  Inputs=2
  Trigonometric Function : Trigonometry  Operator=cos
  Trigonometric Function1 : Trigonometry
  Trigonometric Function2 : Trigonometry
  Trigonometric Function3 : Trigonometry  Operator=cos
  Unary Minus : UnaryMinus
  y1 : Outport
  y2 : Outport  Port=2
  wires:
  Trigonometric Function2/1 -> Mux2/1
  Unary Minus/1 -> Mux1/2
  Trigonometric Function3/1 -> Mux2/2
  Trigonometric Function1/1 -> Unary Minus/1
  alpha/1 -> Trigonometric Function3/1, Trigonometric Function2/1, Trigonometric Function1/1, Trigonometric Function/1
  Mux1/1 -> Dot Product/2
  x1/1 -> Mux/1
  Dot Product1/1 -> y2/1
  Mux2/1 -> Dot Product1/2
  Dot Product/1 -> y1/1
  Mux/1 -> Dot Product1/1, Dot Product/1
  x2/1 -> Mux/2
  Trigonometric Function/1 -> Mux1/1

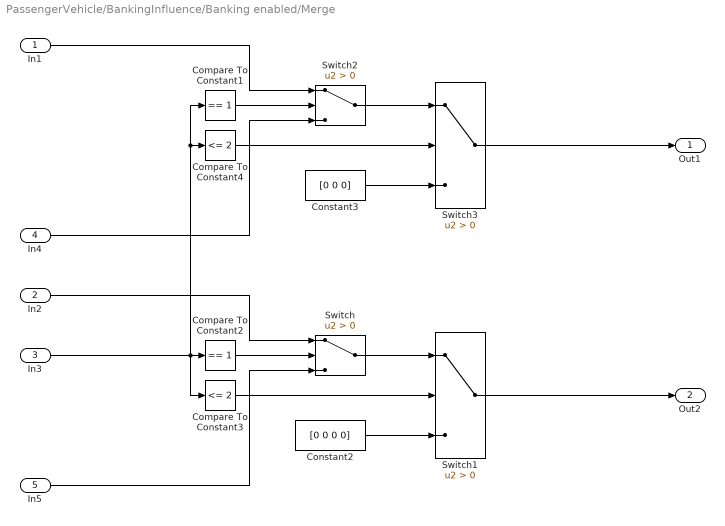
== system PassengerVehicle/BankingInfluence/Banking enabled/Merge ==
  In1 : Inport
  In2 : Inport  Port=2
  In3 : Inport  Port=3
  In4 : Inport  Port=4
  In5 : Inport  Port=5
  Compare To Constant1 : simulink/Logic and Bit Operations/Compare To Constant  relop===  const=1  OutDataTypeStr=boolean
  Compare To Constant2 : simulink/Logic and Bit Operations/Compare To Constant  relop===  const=1  OutDataTypeStr=boolean
  Compare To Constant3 : simulink/Logic and Bit Operations/Compare To Constant  relop=<=  const=2  OutDataTypeStr=boolean
  Compare To Constant4 : simulink/Logic and Bit Operations/Compare To Constant  relop=<=  const=2  OutDataTypeStr=boolean
  Constant2 : Constant  Value=[0 0 0 0]
  Constant3 : Constant  Value=[0 0 0]
  Switch{,1..3} (4 alike) : Switch  Criteria=u2 > Threshold
  Out1 : Outport
  Out2 : Outport  Port=2
  wires:
  In2/1 -> Switch/1
  Compare To Constant2/1 -> Switch/2
  Switch/1 -> Switch1/1
  In5/1 -> Switch/3
  Compare To Constant3/1 -> Switch1/2
  Switch1/1 -> Out2/1
  Constant2/1 -> Switch1/3
  Switch3/1 -> Out1/1
  Constant3/1 -> Switch3/3
  Compare To Constant4/1 -> Switch3/2
  In3/1 -> Compare To Constant3/1, Compare To Constant1/1, Compare To Constant4/1, Compare To Constant2/1
  In4/1 -> Switch2/3
  Switch2/1 -> Switch3/1
  Compare To Constant1/1 -> Switch2/2
  In1/1 -> Switch2/1

== system PassengerVehicle/BankingInfluence/Banking enabled/banking_ndtm ==
  SimRealState : Inport
  Enable : EnablePort
  Bus Selector : BusSelector  OutputSignals=x_m,y_m,psi_rad,ay_mps2
  Constant : Constant  Value=activate_TrackProfile
  Model : ModelReference  ModelNameDialog=banking_ndtm.slx  SimulationMode=Normal  ModelReferenceVersion=1.26
  Mux : Mux  Inputs=3
  TrackPosition : MATLAB Function  TreatAsAtomicUnit=on
  F_K_Extern_N : Outport
  z_I_Ground_m : Outport  Port=2
  wires:
  SimRealState/1 -> Bus Selector/1
  Bus Selector/1 -> Mux/1  "<x_m>"
  Bus Selector/3 -> Mux/3  "<psi_rad>"
  Bus Selector/2 -> Mux/2  "<y_m>"
  TrackPosition/4(info) -> Model/4
  TrackPosition/1(relative_yaw_angle_rad) -> Model/1
  Model/1 -> F_K_Extern_N/1
  Bus Selector/4 -> Model/5  "<ay_mps2>"
  Mux/1 -> TrackPosition/1(States)
  TrackPosition/2(banking_rad) -> Model/2
  Constant/1 -> Model/6
  Model/2 -> z_I_Ground_m/1
  TrackPosition/3(index) -> Model/3

== system PassengerVehicle/BankingInfluence/Banking enabled/banking_nstm ==
  SimRealState : Inport
  Enable : EnablePort
  Bus Selector : BusSelector  OutputSignals=x_m,y_m,psi_rad,ay_mps2
  Constant : Constant  Value=activate_TrackProfile
  Model : ModelReference  ModelNameDialog=banking_nstm.slx  SimulationMode=Normal  ModelReferenceVersion=1.18
  Mux : Mux  Inputs=3
  TrackPosition : MATLAB Function  TreatAsAtomicUnit=on
  F_K_Extern_N : Outport
  z_I_Ground_m : Outport  Port=2
  wires:
  TrackPosition/3(index) -> Model/3
  Model/2 -> z_I_Ground_m/1
  Constant/1 -> Model/6
  TrackPosition/2(banking_rad) -> Model/2
  Mux/1 -> TrackPosition/1(States)
  Bus Selector/4 -> Model/5  "<ay_mps2>"
  Model/1 -> F_K_Extern_N/1
  TrackPosition/1(relative_yaw_angle_rad) -> Model/1
  TrackPosition/4(info) -> Model/4
  Bus Selector/2 -> Mux/2  "<y_m>"
  Bus Selector/3 -> Mux/3  "<psi_rad>"
  Bus Selector/1 -> Mux/1  "<x_m>"
  SimRealState/1 -> Bus Selector/1

== matlab function PassengerVehicle/FrictionInfluence/FrictionInfluence ==
  data: States input; lambda_mue_x output size=[1, 4]; tpa_map input; interpTime input; tpa_map_mode input; lambda_mue_y output size=[1, 4]; Time input
function [lambda_mue_x, lambda_mue_y] = fcn(States, tpa_map, interpTime, tpa_map_mode, Time)

[lambda_mue_x, lambda_mue_y] = FrictionInfluence(States, tpa_map, interpTime, tpa_map_mode, Time);

== matlab function PassengerVehicle/FrictionInfluence/ContactPatchPos ==
  data: States input; States_Tires output; VEH__VehicleData__l_WheelbaseF_m parameter; VEH__VehicleData__l_WheelbaseTotal_m parameter; VEH__VehicleData__w_TrackF_m parameter; VEH__VehicleData__w_TrackR_m parameter
function States_Tires = fcn(States, ...
    VEH__VehicleData__l_WheelbaseF_m, VEH__VehicleData__l_WheelbaseTotal_m, ...
VEH__VehicleData__w_TrackF_m, VEH__VehicleData__w_TrackR_m)

States_Tires = ContactPatchPos(States, ...
    VEH__VehicleData__l_WheelbaseF_m, VEH__VehicleData__l_WheelbaseTotal_m, ...
    VEH__VehicleData__w_TrackF_m, VEH__VehicleData__w_TrackR_m);

== matlab function PassengerVehicle/SensorModels/MATLAB Function ==
  data: u input; y output
function y = normalizeAngle_wrapper(u)

y = normalizeAngle(u);

== matlab function PassengerVehicle/SensorModels/MATLAB Function2 ==
  data: u input; y output
function y = normalizeAngle_wrapper(u)

y = normalizeAngle(u);

== matlab function PassengerVehicle/BankingInfluence/Banking enabled/banking_nstm/TrackPosition ==
  data: Racetrack parameter; States input; relative_yaw_angle_rad output; banking_rad output; index output; info output
function [relative_yaw_angle_rad, banking_rad, index, info] = fcn(Racetrack, States)

[relative_yaw_angle_rad, banking_rad, index, info] = TrackPosition(Racetrack, States);

== matlab function PassengerVehicle/BankingInfluence/Banking enabled/banking_ndtm/TrackPosition ==
  data: Racetrack parameter; States input; relative_yaw_angle_rad output; banking_rad output; index output; info output
function [relative_yaw_angle_rad, banking_rad, index, info] = fcn(Racetrack, States)

[relative_yaw_angle_rad, banking_rad, index, info] = TrackPosition(Racetrack, States);
